simulink model "FinalModel_delF"  (R2021b)
settings: Solver=ode23t  StartTime=0.0  StopTime=4  FixedStep=0.1  RelTol=1e-3
values from neighbouring files (symbols this model uses):
  a = 0.6215    [Constant_Params.m]    (also in HIghSpeedMatlabFile.m = 0.65; RearSteer_SideSlipMin.m = 0.7)
  b = 0.5085    [Constant_Params.m]    (also in HIghSpeedMatlabFile.m = 0.6; RearSteer_SideSlipMin.m = 0.62)
  Cf = 33000    [Constant_Params.m]    (also in HIghSpeedMatlabFile.m = 89.892; RearSteer_SideSlipMin.m = 89.892)
  Cr = 34000    [Constant_Params.m]    (also in HIghSpeedMatlabFile.m = 89.892; RearSteer_SideSlipMin.m = 89.892)
  Iz = 24.47    [Constant_Params.m]    (also in HIghSpeedMatlabFile.m = 194.35)
  L = a+b    (= 1.13)    [Constant_Params.m]    (also in HIghSpeedMatlabFile.m = 1.525)
  m = 230    [Constant_Params.m]    (also in HIghSpeedMatlabFile.m; RearSteer_SideSlipMin.m)
libraries: slpidlib x3, simulink x1, cstblocks x1
settings Model: Creator=Hp  LastModifiedBy=Hp
settings DebuggingCC: AlgebraicLoopMsg=none

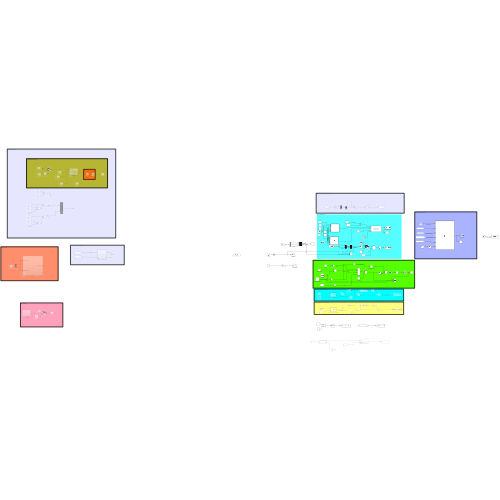
[thumbnail: Simulink's stored preview of the top-level diagram]
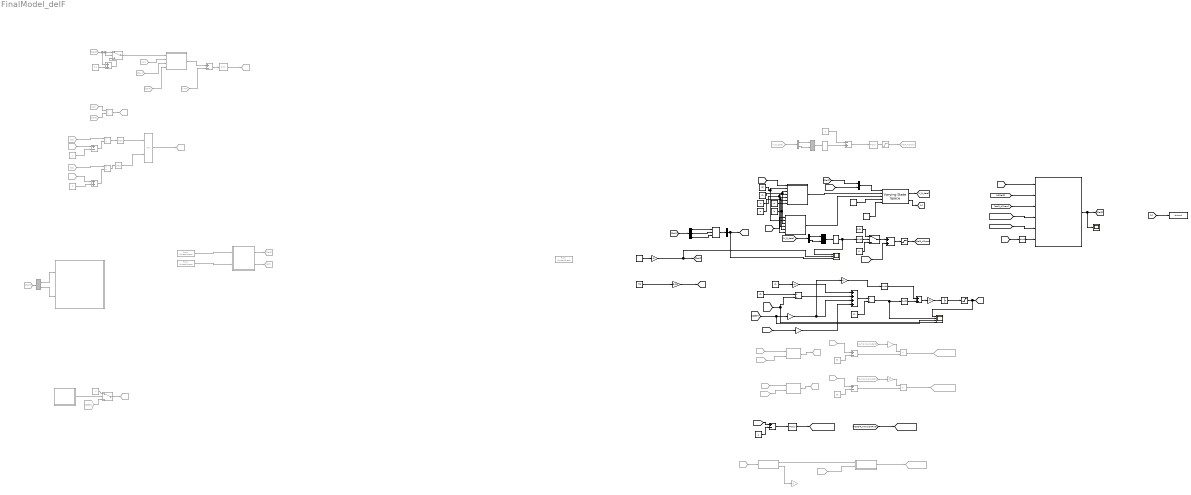
== system FinalModel_delF ==
  note: Switch Data
  note: Vehicle Model
  note: Front Steering Conversion
  note: Low Speed Cornering
  note: Low Speed Cornering Transient
  note: PID Alternative of High Speed Steer
  note: Commented Area
  note: High Speed Cornering
  note: Steering Angle Selector
  note: PID Area
  note: High Speed New
  note: High Speed Cornering Transient
  -2*Cr : Gain  Gain=2*Cr
  -m : Gain  Gain=-m
  0.17*g : Constant  Value=0.17*9.8
  2*Cf+2*Cr : Constant  Value=2*Cf+2*Cr
  2*b*Cr-2*a*Cf : Constant  Value=2*b*Cr-2*a*Cf
  Add : Sum  Inputs=++++
  Add1 : Sum
  Add2 : Sum  Commented=on
  Add3 : Sum  Commented=on  Inputs=+-
  Add4 : Sum  Commented=on  Inputs=+-
  Add5 : Sum  Commented=on
  Add6 : Sum  Commented=on  Inputs=+-
  Add7 : Sum
  Add8 : Sum  Commented=on  Inputs=-+
  Analytical : Subsystem  Commented=on
  Bus Creator : BusCreator  Inputs=2
  Bus Creator1 : BusCreator  Commented=on  Inputs=2
  Bus Creator2 : BusCreator  Inputs=3
  Bus Selector : BusSelector  OutputSignals=yaw rate
  Bus Selector1 : BusSelector  Commented=on  OutputSignals=signal1
  Bus Selector2 : BusSelector  OutputSignals=delR
  Constant : Constant  Commented=on  Value=-7
  Constant1 : Constant  Commented=on  Value=0.1
  Constant10 : Constant  Value=Cr
  Constant11 : Constant  Value=Iz
  Constant12 : Constant  Value=a
  Constant13 : Constant  Value=b
  Constant14 : Constant  Value=m
  Constant15 : Constant  Value=56
  Constant18 : Constant
  Constant2 : Constant  Commented=on  Value=35
  Constant3 : Constant  Commented=on  Value=35
  Constant4 : Constant  Value=[0 0;0 0]
  Constant5 : Constant  Value=[1 0;0 1]
  Constant6 : Constant  Value=0.01
  Constant7 : Constant  Value=0
  Constant8 : Constant  Commented=on  Value=0
  Constant9 : Constant  Value=Cf
  DelFront Derivative : Derivative
  DelRSwitch : Goto  Commented=on  GotoTag=DelRSwitch
  Demux : Demux  Commented=on  Outputs=2
  Demux1 : Demux  Outputs=2
  Demux2 : Demux  Commented=on  Outputs=2
  Demux3 : Demux  Outputs=3
  Derivative : Derivative
  Derivative1 : Derivative
  Derivative2 : Derivative
  Divide : Product  Inputs=*/
  Divide1 : Product  Inputs=*/
  Divide2 : Product  Commented=on  Inputs=**
  Divide3 : Product  Commented=on  Inputs=**
  Divide4 : Product  Commented=on  Inputs=*/
  Divide5 : Product  Commented=on  Inputs=*/
  Divide6 : Product  Commented=on  Inputs=*/
  From : From  Commented=on  GotoTag=DelR
  From Spreadsheet : FromSpreadsheet  Commented=on  FileName=D:\Transfer_Files\IIT_RMS\Vehicle Dynamics\Rear Steering\Steering Geometry section\Final MOdel\del_if.xlsx  Range=B1:B100  TreatFirstColumnAs=Data
  From Spreadsheet1 : FromSpreadsheet  Commented=on  FileName=D:\Transfer_Files\IIT_RMS\Vehicle Dynamics\Rear Steering\Steering Geometry section\Final MOdel\del_of.xlsx  SheetName=Sheet 1  Range=B1:B100
  From Spreadsheet2 : FromSpreadsheet  Commented=on  FileName=delF.xlsx  SheetName=Sheet2  Range=A1:A355  TreatFirstColumnAs=Data
  From1 : From  Commented=on  GotoTag=DelR
  From{10,12,14,16,40} (5 alike) : From  Commented=on  GotoTag=Velocity
  From11 : From  Commented=on  GotoTag=Bi_delR
  From13 : From  Commented=on  GotoTag=C2
  From17 : From  Commented=on  GotoTag=DelR
  From18 : From  Commented=on  GotoTag=HS_Transient_delR
  From2 : From  Commented=on  GotoTag=YAW
  From23 : From  Commented=on  GotoTag=C2
  From24 : From  Commented=on  GotoTag=Rrear
  From25 : From  Commented=on  GotoTag=C2
  From26 : From  Commented=on  GotoTag=Rrear
  From3 : From  Commented=on  GotoTag=Ay
  From33 : From  Commented=on  GotoTag=V_R_data
  From37 : From  Commented=on  GotoTag=Bi_delR
  From39 : From  Commented=on  GotoTag=Bi_delR
  From4 : From  Commented=on  GotoTag=RAy
  From5 : From  Commented=on  GotoTag=DelF
  From9 : From  Commented=on  GotoTag=LS_Transient_delR
  Front Steer : Goto  Commented=on  GotoTag=DelF
  Gain : Gain  Gain=-1*(Cf+Cr)/Cr
  Gain1 : Gain  Gain=2*Cf
  Gain2 : Gain  Gain=1/(2*Cf+2*Cr)
  Gain3 : Gain  Commented=on  Gain=-1/2
  Gain4 : Gain  Commented=on  Gain=1/2
  Gain5 : Gain  Gain=3.14'/180
  Gain6 : Gain  Commented=on  Gain=0
  Gain8 : Gain  Gain=5/18
  Goto1 : Goto  Commented=on  GotoTag=delR_HSnew
  Goto12 : Goto  Commented=on  GotoTag=LSDelR_TransientFinal
  Goto4 : Goto  Commented=on  GotoTag=LSDelR_TransientFinal
  Goto5 : Goto  Commented=on  GotoTag=HSDelR_TransientFinal
  Goto6 : Goto  Commented=on  GotoTag=delR_Combined
  High Speed Transint Function : MATLAB Function  Commented=on  TreatAsAtomicUnit=on
  If1 : If  Commented=on  IfExpression=u1 <=35 & u1>33
  Integrator : Integrator
  Low Speed DelR Transient : Goto  Commented=on  GotoTag=LS_Transient_delR
  Low Speed DelR Transient1 : Goto  Commented=on  GotoTag=HS_Transient_delR
  Low Speed Transient Function : MATLAB Function  Commented=on  TreatAsAtomicUnit=on
  MATLAB Function : MATLAB Function  TreatAsAtomicUnit=on
  MATLAB Function1 : MATLAB Function  TreatAsAtomicUnit=on
  MATLAB Function2 : MATLAB Function  TreatAsAtomicUnit=on
  Mux : Mux  Commented=on  Inputs=2
  Mux1 : Mux  Inputs=2
  PID Controller : slpidlib/PID Controller  Commented=on  Controller=PI  Form=Parallel  TimeDomain=Continuous-time  UseExternalTs=off  SampleTime=-1  IntegratorMethod=Forward Euler  FilterMethod=Forward Euler  ControllerParametersSource=internal  P=1  I=1  D=0  UseFilter=on  N=100  TunerSelectOption=Transfer Function Based (PID Tuner App)  InitialConditionSource=internal  InitialConditionForIntegrator=0  InitialConditionForFilter=0  DifferentiatorICPrevScaledInput=0  ExternalReset=none  TrackingMode=off  Kt=1  LimitOutput=on  SatLimitsSource=internal  UpperSaturationLimit=6  LowerSaturationLimit=-6  LinearizeAsGain=on  AntiWindupMode=none  Kb=1  POutMin=[]  POutMax=[]  IOutMin=[]  IOutMax=[]  DOutMin=[]  DOutMax=[]  NOutMin=[]  NOutMax=[]  SumOutMin=[]  SumOutMax=[]  SaturationOutMin=[]  SaturationOutMax=[]  PParamMin=[]  PParamMax=[]  IParamMin=[]  IParamMax=[]  DParamMin=[]  DParamMax=[]  NParamMin=[]  NParamMax=[]  KbParamMin=[]  KbParamMax=[]  KtParamMin=[]  KtParamMax=[]  KbOutMin=[]  KbOutMax=[]  KtOutMin=[]  KtOutMax=[]  IntegratorOutMin=[]  IntegratorOutMax=[]  FilterOutMin=[]  FilterOutMax=[]  SumI1OutMin=[]  SumI1OutMax=[]  SumI2OutMin=[]  SumI2OutMax=[]  SumI3OutMin=[]  SumI3OutMax=[]  SumI4OutMin=[]  SumI4OutMax=[]  SumDOutMin=[]  SumDOutMax=[]  DifferentiatorOutMin=[]  DifferentiatorOutMax=[]  FilterDiffOutCoefMin=[]  FilterDiffOutCoefMax=[]  ReciprocalOutMin=[]  ReciprocalOutMax=[]  SumDenOutMin=[]  SumDenOutMax=[]  SumNumOutMin=[]  SumNumOutMax=[]  DivideOutMin=[]  DivideOutMax=[]  UdiffTsProdOutMin=[]  UdiffTsProdOutMax=[]  NTsProdOutMin=[]  NTsProdOutMax=[]  UintegralTsProdOutMin=[]  UintegralTsProdOutMax=[]  UngainTsProdOutMin=[]  UngainTsProdOutMax=[]  IntegratorContinuousStateAttributes=''  IntegratorStateMustResolveToSignalObject=off  IntegratorRTWStateStorageClass=Auto  FilterContinuousStateAttributes=''  FilterStateMustResolveToSignalObject=off  FilterRTWStateStorageClass=Auto  ParallelPVariant=InternalParameters  IdealPVariant=Disabled  IVariant=InternalParameters  DVariant=Disabled  IntegratorVariant=Continuous  SatVariant=Enabled  AWVariant=Passthrough  PCopyVariant=Disabled  TRVariant=Disabled  FdbkBlocksVariant=Forward  IdealPFdbkVariant=Disabled  SatFdbkVariant=Disabled  DerivativeFilterVariant=Disabled  NVariant=Disabled  NCopyVariant=Disabled_SignalSpec  FilterICVariant=Disabled  IntegratorICVariant=InternalICs  ExternalResetVariant=Disabled  TRSumVariant=Passthrough  SumFdbkVariant=Disabled  SumVariant=Sum_PI  TsampFilterVariant=InternalTs  TsampNgainVariant=Passthrough  TsampIntegralVariant=Passthrough  ExternalSaturationOutDataTypeStr=Inherit: Same as second input
  PID Controller1 : slpidlib/PID Controller  Commented=on  Controller=PID  Form=Parallel  TimeDomain=Continuous-time  UseExternalTs=off  SampleTime=-1  IntegratorMethod=Forward Euler  FilterMethod=Forward Euler  ControllerParametersSource=internal  P=1  I=1  D=0  UseFilter=on  N=100  TunerSelectOption=Transfer Function Based (PID Tuner App)  InitialConditionSource=internal  InitialConditionForIntegrator=0  InitialConditionForFilter=0  DifferentiatorICPrevScaledInput=0  ExternalReset=none  TrackingMode=off  Kt=1  LimitOutput=off  SatLimitsSource=internal  UpperSaturationLimit=inf  LowerSaturationLimit=-inf  LinearizeAsGain=on  AntiWindupMode=none  Kb=1  POutMin=[]  POutMax=[]  IOutMin=[]  IOutMax=[]  DOutMin=[]  DOutMax=[]  NOutMin=[]  NOutMax=[]  SumOutMin=[]  SumOutMax=[]  SaturationOutMin=[]  SaturationOutMax=[]  PParamMin=[]  PParamMax=[]  IParamMin=[]  IParamMax=[]  DParamMin=[]  DParamMax=[]  NParamMin=[]  NParamMax=[]  KbParamMin=[]  KbParamMax=[]  KtParamMin=[]  KtParamMax=[]  KbOutMin=[]  KbOutMax=[]  KtOutMin=[]  KtOutMax=[]  IntegratorOutMin=[]  IntegratorOutMax=[]  FilterOutMin=[]  FilterOutMax=[]  SumI1OutMin=[]  SumI1OutMax=[]  SumI2OutMin=[]  SumI2OutMax=[]  SumI3OutMin=[]  SumI3OutMax=[]  SumI4OutMin=[]  SumI4OutMax=[]  SumDOutMin=[]  SumDOutMax=[]  DifferentiatorOutMin=[]  DifferentiatorOutMax=[]  FilterDiffOutCoefMin=[]  FilterDiffOutCoefMax=[]  ReciprocalOutMin=[]  ReciprocalOutMax=[]  SumDenOutMin=[]  SumDenOutMax=[]  SumNumOutMin=[]  SumNumOutMax=[]  DivideOutMin=[]  DivideOutMax=[]  UdiffTsProdOutMin=[]  UdiffTsProdOutMax=[]  NTsProdOutMin=[]  NTsProdOutMax=[]  UintegralTsProdOutMin=[]  UintegralTsProdOutMax=[]  UngainTsProdOutMin=[]  UngainTsProdOutMax=[]  IntegratorContinuousStateAttributes=''  IntegratorStateMustResolveToSignalObject=off  IntegratorRTWStateStorageClass=Auto  FilterContinuousStateAttributes=''  FilterStateMustResolveToSignalObject=off  FilterRTWStateStorageClass=Auto  ParallelPVariant=InternalParameters  IdealPVariant=Disabled  IVariant=InternalParameters  DVariant=InternalParameters  IntegratorVariant=Continuous  SatVariant=Disabled  AWVariant=Passthrough  PCopyVariant=Disabled  TRVariant=Disabled  FdbkBlocksVariant=Forward  IdealPFdbkVariant=Disabled  SatFdbkVariant=Disabled  DerivativeFilterVariant=ContFilter  NVariant=InternalParameters  NCopyVariant=Disabled  FilterICVariant=InternalICsFilter  IntegratorICVariant=InternalICs  ExternalResetVariant=Disabled  TRSumVariant=Passthrough  SumFdbkVariant=Disabled  SumVariant=Sum_PID  TsampFilterVariant=InternalTs  TsampNgainVariant=Passthrough  TsampIntegralVariant=Passthrough  ExternalSaturationOutDataTypeStr=Inherit: Same as second input
  PID Controller2 : slpidlib/PID Controller  Controller=PID  Form=Parallel  TimeDomain=Continuous-time  UseExternalTs=off  SampleTime=-1  IntegratorMethod=Forward Euler  FilterMethod=Forward Euler  ControllerParametersSource=internal  P=1  I=1  D=0  UseFilter=on  N=100  TunerSelectOption=Transfer Function Based (PID Tuner App)  InitialConditionSource=internal  InitialConditionForIntegrator=0  InitialConditionForFilter=0  DifferentiatorICPrevScaledInput=0  ExternalReset=none  TrackingMode=off  Kt=1  LimitOutput=off  SatLimitsSource=internal  UpperSaturationLimit=inf  LowerSaturationLimit=-inf  LinearizeAsGain=on  AntiWindupMode=none  Kb=1  POutMin=[]  POutMax=[]  IOutMin=[]  IOutMax=[]  DOutMin=[]  DOutMax=[]  NOutMin=[]  NOutMax=[]  SumOutMin=[]  SumOutMax=[]  SaturationOutMin=[]  SaturationOutMax=[]  PParamMin=[]  PParamMax=[]  IParamMin=[]  IParamMax=[]  DParamMin=[]  DParamMax=[]  NParamMin=[]  NParamMax=[]  KbParamMin=[]  KbParamMax=[]  KtParamMin=[]  KtParamMax=[]  KbOutMin=[]  KbOutMax=[]  KtOutMin=[]  KtOutMax=[]  IntegratorOutMin=[]  IntegratorOutMax=[]  FilterOutMin=[]  FilterOutMax=[]  SumI1OutMin=[]  SumI1OutMax=[]  SumI2OutMin=[]  SumI2OutMax=[]  SumI3OutMin=[]  SumI3OutMax=[]  SumI4OutMin=[]  SumI4OutMax=[]  SumDOutMin=[]  SumDOutMax=[]  DifferentiatorOutMin=[]  DifferentiatorOutMax=[]  FilterDiffOutCoefMin=[]  FilterDiffOutCoefMax=[]  ReciprocalOutMin=[]  ReciprocalOutMax=[]  SumDenOutMin=[]  SumDenOutMax=[]  SumNumOutMin=[]  SumNumOutMax=[]  DivideOutMin=[]  DivideOutMax=[]  UdiffTsProdOutMin=[]  UdiffTsProdOutMax=[]  NTsProdOutMin=[]  NTsProdOutMax=[]  UintegralTsProdOutMin=[]  UintegralTsProdOutMax=[]  UngainTsProdOutMin=[]  UngainTsProdOutMax=[]  IntegratorContinuousStateAttributes=''  IntegratorStateMustResolveToSignalObject=off  IntegratorRTWStateStorageClass=Auto  FilterContinuousStateAttributes=''  FilterStateMustResolveToSignalObject=off  FilterRTWStateStorageClass=Auto  ParallelPVariant=InternalParameters  IdealPVariant=Disabled  IVariant=InternalParameters  DVariant=InternalParameters  IntegratorVariant=Continuous  SatVariant=Disabled  AWVariant=Passthrough  PCopyVariant=Disabled  TRVariant=Disabled  FdbkBlocksVariant=Forward  IdealPFdbkVariant=Disabled  SatFdbkVariant=Disabled  DerivativeFilterVariant=ContFilter  NVariant=InternalParameters  NCopyVariant=Disabled  FilterICVariant=InternalICsFilter  IntegratorICVariant=InternalICs  ExternalResetVariant=Disabled  TRSumVariant=Passthrough  SumFdbkVariant=Disabled  SumVariant=Sum_PID  TsampFilterVariant=InternalTs  TsampNgainVariant=Passthrough  TsampIntegralVariant=Passthrough  ExternalSaturationOutDataTypeStr=Inherit: Same as second input
  Ramp : simulink/Sources/Ramp  slope=20  start=0  InitialOutput=0
  Rear Steer : Goto  Commented=on  GotoTag=HSDelR
  Rear track : Constant  Commented=on
  Rear track1 : Constant  Commented=on
  Rrear : Goto  Commented=on  GotoTag=Rrear
  Saturation : Saturate  UpperLimit=6  LowerLimit=-6  LinearizeAsGain=off  ZeroCross=off  RndMeth=Ceiling
  Saturation1 : Saturate  UpperLimit=6*(3.14/180)  LowerLimit=-6*(3.14/180)
  Saturation2 : Saturate  Commented=on  UpperLimit=6  LowerLimit=-6
  Scope : Scope  NumInputPorts=4
  Scope1 : Scope
  Scope2 : Scope  NumInputPorts=3
  Subsystem : Subsystem  Commented=on
  Subsystem2 : Subsystem  Commented=on
  Subtract : Sum  Commented=on  Inputs=+-
  Subtract1 : Sum  Inputs=+-
  Switch : Switch  Commented=on  Criteria=u2 ~= 0
  Switch Data : Subsystem  Commented=on
  Switch1 : Switch  Criteria=u2 > Threshold
  Switch2 : Switch  Commented=on  Criteria=u2 ~= 0
  Tan : Trigonometry  Commented=on  Operator=atan
  Tan1 : Trigonometry  Commented=on  Operator=atan
  To Workspace : ToWorkspace  VariableName=simout  SaveFormat=Timeseries  SampleTime=-1
  Varying State Space : cstblocks/Linear Parameter Varying/Varying State Space  x0=0  xNames=''  OutputX=on  OutputDX=off
  Vehicle : Subsystem  Commented=on
  Velocity1 : From  Commented=on  GotoTag=DelR
  c2 : Goto  Commented=on  GotoTag=C2
  wires:
  Constant9/1 -> MATLAB Function1/2(Cf), MATLAB Function2/2(Cf)
  Saturation2/1 -> Goto1/1
  [Bi_delR] -> Subtract1/1
  [DelR] -> Demux3/1  "del_R"
  If1/1 -> Subsystem2/1(Velocity)
  Constant12/1 -> MATLAB Function2/4(a), MATLAB Function1/5(a)
  Bus Selector2/1 -> Scope2/3, [Bi_delR]  "<delR>"
  Subtract1/1 -> PID Controller2/1
  PID Controller2/1 -> [HSDelR_TransientFinal]
  -m/1 -> Add/1  "-m*ay"
  Demux2/2 -> Bus Creator1/2
  Constant3/1 -> Add6/2
  Subsystem2/1(Out1) -> Goto12/1
  Constant10/1 -> MATLAB Function2/3(Cr), MATLAB Function1/3(Cr)
  From/1 -> Add2/1, Switch/2, Switch/1
  Bus Selector1/1 -> Add8/2  "<signal1>"
  [Velocity] -> MATLAB Function1/1(u)
  High Speed Transint Function/1(y) -> Low Speed DelR Transient1/1
  Bus Creator1/1 -> Bus Selector1/1
  MATLAB Function1/1(y) -> Varying State Space/2
  Demux3/1 -> Bus Creator2/1
  From39/1 -> Subsystem2/2(Bi_delR)
  Constant18/1 -> Subtract1/2
  -2*Cr/1 -> Add/4  "2*C"
  Subsystem/2(C2) -> c2/1
  Mux1/1 -> Varying State Space/1
  Demux1/1 -> Bus Creator/1
  Constant14/1 -> MATLAB Function1/7(m)
  Derivative1/1 -> MATLAB Function/6(der)
  From13/1 -> Divide4/1
  From9/1 -> Gain3/1
  Divide5/1 -> Tan/1
  Demux3/3 -> Bus Creator2/3  "delR"
  Bus Creator2/1 -> Bus Selector2/1
  Demux/2 -> Vehicle/2(Outer Wheel Steer)
  Demux2/1 -> Bus Creator1/1
  Constant8/1 -> Add8/1
  [Bi_delR] -> -2*Cr/1
  Derivative2/1 -> Switch1/2
  Switch/1 -> Analytical/1(Rear steer)  "Del R"
  Add7/1 -> Saturation1/1
  Constant7/1 -> Switch1/3
  PID Controller1/1 -> Saturation2/1
  From33/1 -> Demux2/1
  Switch2/1 -> DelRSwitch/1
  Subsystem/1(Out1) -> Front Steer/1
  From25/1 -> Divide6/1
  Saturation1/1 -> [delR_HSnew]
  Constant11/1 -> MATLAB Function1/4(Iz), MATLAB Function2/6(Iz)
  [Velocity] -> MATLAB Function/1(u)  "Vehicle Velocity"
  [Bi_delR] -> Add7/2  "del_R"
  Bus Creator/1 -> Bus Selector/1
  Low Speed Transient Function/1(y) -> Low Speed DelR Transient/1
  Switch1/1 -> Add7/1
  Constant/1 -> Switch2/1
  Constant6/1 -> Switch1/1
  From1/1 -> Demux/1
  From18/1 -> Gain4/1
  From23/1 -> Divide5/1
  Varying State Space/1 -> [V_R_data]
  [Velocity] -> Derivative1/1
  Divide6/1 -> Tan1/1
  Add1/1 -> Gain/1
  MATLAB Function2/1(y) -> Varying State Space/3
  [LSDelR_TransientFinal] -> MATLAB Function/4(LsT)  "Low Speed Transient"
  Varying State Space/2 -> [x]
  Divide2/1 -> Goto4/1  "delR Low Speed Transient"
  Bus Selector/1 -> Scope2/1, Derivative2/1  "<yaw rate>"
  Demux1/2 -> Bus Creator/2  "yaw rate"
  [V_R_data] -> Demux1/1
  DelFront Derivative/1 -> Add1/1
  Integrator/1 -> Saturation/1  "Rear Steer"
  Demux/1 -> Vehicle/1(Inner Wheel Steer)
  Constant5/1 -> Varying State Space/4
  [Velocity] -> MATLAB Function2/1(u)
  [DelF] -> Mux1/1  "del_F"
  Add4/1 -> Divide2/2
  From2/1 -> Subtract/2
  Add6/1 -> Divide3/2
  Divide3/1 -> Goto5/1  "delR Low Speed Transient"
  From26/1 -> Add5/1
  Tan1/1 -> Mux/2
  Rear track1/1 -> Add5/2
  From Spreadsheet1/1 -> Subsystem/2(In2)  "del Outer"
  Add3/1 -> Divide5/2
  Divide4/1 -> Rrear/1
  [Bi_delR] -> Mux1/2
  Tan/1 -> Mux/1
  Demux3/2 -> Bus Creator2/2
  Mux/1 -> Goto6/1
  From14/1 -> High Speed Transint Function/1(u)
  Gain2/1 -> DelFront Derivative/1  "2*Cf*delfront/(2Cf+Cr)"
  From17/1 -> Divide4/2
  [delR_HSnew] -> MATLAB Function/3(Hs)  "High Speed Steering"
  MATLAB Function/1(y) -> [DelR], Scope1/1
  From4/1 -> Analytical/3(Rear Lateral Accelation)  "Rear Ay"
  From10/1 -> Low Speed Transient Function/1(u)
  Add5/1 -> Divide6/2
  Gain3/1 -> Divide2/1
  From16/1 -> Add6/1
  Subtract/1 -> PID Controller/1
  Constant2/1 -> Add4/2
  If1/2 -> Gain6/1
  [LSDelR] -> MATLAB Function/2(Ls)  "Low Speed Steering"
  Switch Data/1(Out1) -> Switch2/2
  Constant13/1 -> MATLAB Function1/6(b), MATLAB Function2/5(b)
  From Spreadsheet/1 -> Subsystem/1(In1)  "del Inner"
  From24/1 -> Add3/1
  From3/1 -> Analytical/2(Lateral Acceleration)  "Ay"
  PID Controller/1 -> Rear Steer/1
  Add2/1 -> Switch/3
  Gain1/1 -> Gain2/1, Add/3  "2*Cf*delfront"
  From5/1 -> Analytical/4(Front Steering)  "Ref Model"
  Analytical/1("Omega Analytical ") -> Subtract/1  "Ref Model"
  [DelF] -> Scope/3, Gain1/1  "FrontSteering Input"
  Saturation/1 -> Scope/1, [LSDelR]
  From12/1 -> Add4/1
  Divide1/1 -> Derivative/1, Scope/2  "Side Slip Angle"
  2*Cf+2*Cr/1 -> Divide1/2
  Add8/1 -> PID Controller1/1
  From11/1 -> High Speed Transint Function/2(z)
  Gain/1 -> Integrator/1
  Constant4/1 -> Varying State Space/5
  Constant1/1 -> Add2/2
  Velocity1/1 -> Switch2/3
  Derivative/1 -> Add1/2  "d(Beta)/dt"
  Add/1 -> Divide1/1
  From37/1 -> Low Speed Transient Function/2(z)
  From40/1 -> If1/1
  Divide/1 -> Add/2  "(2*b*Cr-2*a*Cf)/Vx"
  [HSDelR_TransientFinal] -> [LSDelR_TransientFinal]
  [HSDelR_TransientFinal] -> MATLAB Function/5(HsT)  "HIgh Speed Transient"
  Gain4/1 -> Divide3/1
  0.17*g/1 -> -m/1  "ay"
  [Velocity] -> Divide/2, Scope/4
  Rear track/1 -> Add3/2
  2*b*Cr-2*a*Cf/1 -> Divide/1
  Constant15/1 -> Gain8/1
  Gain8/1 -> [Velocity]
  Gain5/1 -> Scope2/2, [DelF]  "delF"
  Ramp/1 -> Gain5/1
  [x] -> To Workspace/1  "Vehicle Velocity"

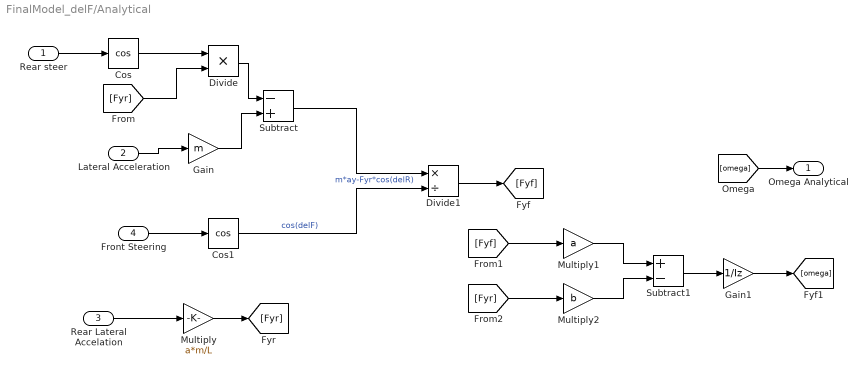
== system FinalModel_delF/Analytical ==
  Rear steer : Inport
  Lateral Acceleration : Inport  Port=2
  Rear Lateral Accelation : Inport  Port=3
  Front Steering : Inport  Port=4
  Cos : Trigonometry  Operator=cos
  Cos1 : Trigonometry  Operator=cos
  Divide : Product  Inputs=**
  Divide1 : Product  Inputs=*/
  Gain : Gain  Gain=m
  Gain1 : Gain  Gain=1/Iz
  Multiply : Gain  Gain=a*m/L
  Multiply1 : Gain  Gain=a
  Multiply2 : Gain  Gain=b
  Subtract : Sum  Inputs=-+
  Subtract1 : Sum  Inputs=+-
  "Omega Analytical " : Outport
  wires:
  Rear Lateral Accelation/1 -> Multiply/1
  Multiply/1 -> [Fyr]
  [omega] -> "Omega Analytical "/1
  Rear steer/1 -> Cos/1
  Front Steering/1 -> Cos1/1
  Cos/1 -> Divide/1
  [Fyr] -> Divide/2
  Divide/1 -> Subtract/1
  Lateral Acceleration/1 -> Gain/1
  Gain/1 -> Subtract/2
  Subtract/1 -> Divide1/1  "m*ay-Fyr*cos(delR)"
  Cos1/1 -> Divide1/2  "cos(delF)"
  Divide1/1 -> [Fyf]
  [Fyf] -> Multiply1/1
  [Fyr] -> Multiply2/1
  Multiply1/1 -> Subtract1/1
  Multiply2/1 -> Subtract1/2
  Subtract1/1 -> Gain1/1
  Gain1/1 -> [omega]

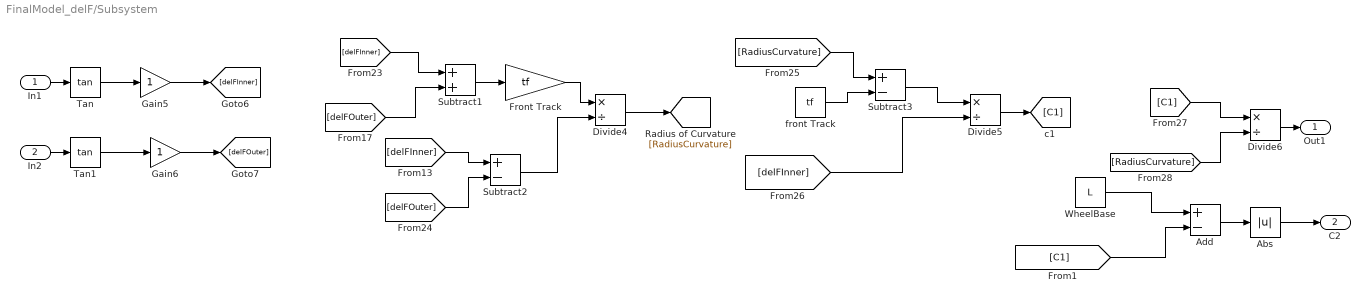
== system FinalModel_delF/Subsystem ==
  In1 : Inport
  In2 : Inport  Port=2
  Abs : Abs
  Add : Sum  Inputs=+-
  Divide4 : Product  Inputs=*/
  Divide5 : Product  Inputs=*/
  Divide6 : Product  Inputs=*/
  Front Track : Gain  Gain=tf
  Gain5 : Gain
  Gain6 : Gain
  Subtract1 : Sum
  Subtract2 : Sum  Inputs=+-
  Subtract3 : Sum  Inputs=+-
  Tan : Trigonometry  Operator=tan
  Tan1 : Trigonometry  Operator=tan
  WheelBase : Constant  Value=L
  front Track : Constant  Value=tf
  Out1 : Outport
  C2 : Outport  Port=2
  wires:
  Subtract1/1 -> Front Track/1
  Gain6/1 -> [delFOuter]
  Divide5/1 -> [C1]
  [delFOuter] -> Subtract2/2
  Subtract3/1 -> Divide5/1
  [delFInner] -> Divide5/2
  [RadiusCurvature] -> Divide6/2
  front Track/1 -> Subtract3/2
  [C1] -> Divide6/1
  Front Track/1 -> Divide4/1
  Subtract2/1 -> Divide4/2
  [delFInner] -> Subtract1/1
  [delFOuter] -> Subtract1/2
  Divide6/1 -> Out1/1
  Divide4/1 -> [RadiusCurvature]
  [delFInner] -> Subtract2/1
  In2/1 -> Tan1/1
  Gain5/1 -> [delFInner]
  Tan/1 -> Gain5/1
  [RadiusCurvature] -> Subtract3/1
  Tan1/1 -> Gain6/1
  In1/1 -> Tan/1
  WheelBase/1 -> Add/1
  [C1] -> Add/2
  Add/1 -> Abs/1
  Abs/1 -> C2/1

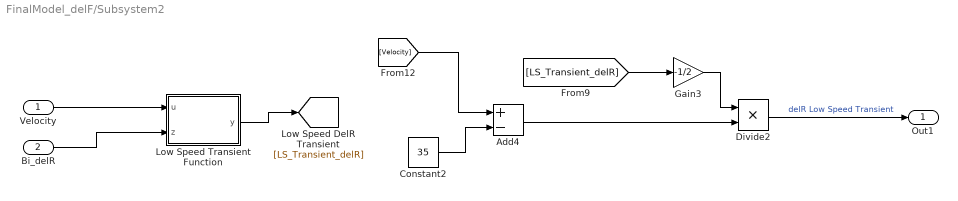
== system FinalModel_delF/Subsystem2 ==
  Velocity : Inport
  Bi_delR : Inport  Port=2
  Add4 : Sum  Inputs=+-
  Constant2 : Constant  Value=35
  Divide2 : Product  Inputs=**
  Gain3 : Gain  Gain=-1/2
  Low Speed Transient Function : MATLAB Function  TreatAsAtomicUnit=on
  Out1 : Outport
  wires:
  Bi_delR/1 -> Low Speed Transient Function/2(z)
  Gain3/1 -> Divide2/1
  Velocity/1 -> Low Speed Transient Function/1(u)
  [LS_Transient_delR] -> Gain3/1
  Add4/1 -> Divide2/2
  [Velocity] -> Add4/1
  Low Speed Transient Function/1(y) -> [LS_Transient_delR]
  Constant2/1 -> Add4/2
  Divide2/1 -> Out1/1  "delR Low Speed Transient"

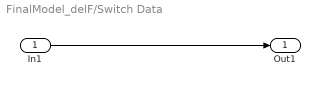
== system FinalModel_delF/Switch Data ==
  In1 : Inport
  Out1 : Outport
  wires:
  In1/1 -> Out1/1

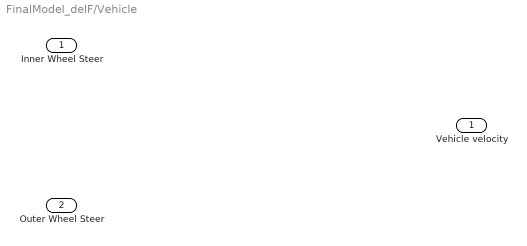
== system FinalModel_delF/Vehicle ==
  Inner Wheel Steer : Inport
  Outer Wheel Steer : Inport  Port=2
  Vehicle velocity : Outport

== matlab function FinalModel_delF/High Speed Transint Function ==
  data: u input; y output; z input
function y = fcn(u,z)

if u==37
    HS_Transient_delR=z;
end

y=HS_Transient_delR;

== matlab function FinalModel_delF/Low Speed Transient Function ==
  data: u input; y output; z input
function y = fcn(u,z)

if u==33
    LS_Transient_delR=z;
else
    LS_Transient_delR=0;
end
    
y=LS_Transient_delR;

== matlab function FinalModel_delF/MATLAB Function ==
  data: u input; y output; Ls input; Hs input; LsT input; HsT input; der input
function y = fcn(u, Ls, Hs, LsT, HsT, der)
%     if Hs==0
%         delr_i=0;
%         delr_o=0;
%     else
% %        delr_i=atan(C2/((C2/Hs)-tf));
% %        delr_o=atan(C2/((C2/Hs)+tf));
%     end    
    if u<(33*5/18)
        %y=[delr_i delr_o Ls];
        y=[Ls Ls Ls];
    elseif u>=(33*5/18) && u<=(35*5/18)
        if der>0
            y=[LsT LsT LsT];
        else 
            y=[Ls Ls Ls];
        end
    elseif  u>(35*5/18) && u<=(37*5/18)
        if der>0
            y=[Hs Hs Hs];
        else 
            y=[HsT HsT HsT];
        end
    else
        y=[Hs Hs Hs];
    end

== matlab function FinalModel_delF/MATLAB Function1 ==
  data: u input; y output; Cf input; Cr input; Iz input; a input; b input; m input
function y = fcn(u,Cf,Cr,Iz,a,b,m)

y = [-(Cf+Cr)/(m*u) ((-a*Cf+b*Cr)/(m*u)-u);-(a*Cf-b*Cr)/(Iz*u) -((a*a*Cf+b*b*Cr)/(Iz*u))];

== matlab function FinalModel_delF/MATLAB Function2 ==
  data: u input; y output; Cf input; Cr input; a input; b input; Iz input
function y = fcn(u,Cf,Cr,a,b,Iz)

y = [Cf/u Cr/u;(a*Cf/Iz) (-b*Cr/Iz)];

== matlab function FinalModel_delF/Subsystem2/Low Speed Transient Function ==
  data: u input; y output; z input
function y = fcn(u,z)

if u==33
    LS_Transient_delR=z;
else
    LS_Transient_delR=0;
end
    
y=LS_Transient_delR;
